simulink model "task1"  (R2017a)
settings: Solver=VariableStepAuto  StartTime=0.0  StopTime=10.0  RelTol=1e-3
libraries: simrfV2elements x2, elec_lib x1
settings Model: Creator=Oskar  LastModifiedBy=Oskar

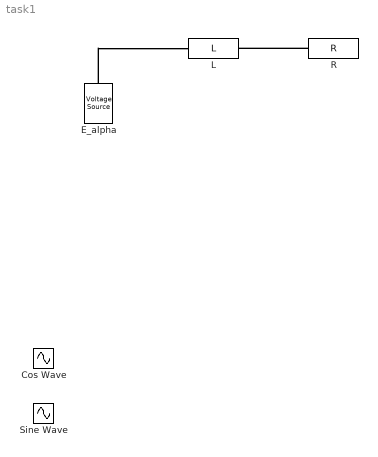
== system task1 ==
  Cos Wave : Sin  Phase=pi/2  SampleTime=0
  E_alpha : elec_lib/Sources/Voltage Source  dc_voltage=0 V  ac_voltage=V_base V  ac_shift=pi/2 rad  ac_frequency=50 Hz  noise_mode=0  PSD=0 V^2/Hz  repeatability=1  auto_seed=4120988592  user_seed=0  sample_time=1e-3 s  i_specify=off  i_priority=None  i=0 A  i_nominal_specify=off  i_nominal_unit=A  i_nominal_value=1  v_specify=off  v_priority=None  v=0 V  v_nominal_specify=off  v_nominal_unit=V  v_nominal_value=1
      settings: SourceProductName=Simscape Electronics  SourceProductBaseCode=SN
  L : simrfV2elements/L  classname=inductor  Inductance=0.2426 H
      settings: SourceProductName=SimRF  SourceProductBaseCode=RB
  R : simrfV2elements/R  classname=resistor  Resistance=0.02 Ohm  AddNoise=on
      settings: SourceProductName=SimRF  SourceProductBaseCode=RB
  Sine Wave : Sin  SampleTime=0
  connections:
  R/LConn1 -- L/RConn1
  E_alpha/LConn1 -- L/LConn1
